simulink model "DebitPapillon_1"  (R2024b)
settings: Solver=FixedStepDiscrete  StartTime=0.0  StopTime=SimuPapStop  FixedStep=0.1  RelTol=1e-3  EnableMultiTasking=on
undefined symbols (not defined in the file): AirIntakeAirFlowTest, AirIntakeTemperatureTest, AirIntakeTimeTest, gam, Pamb, PcolPapTest, PRcrit, Rair, SectionPapTest, Tamb, TempsPapTest
settings Model: Creator=a030141  LastModifiedBy=ramse
settings SolverCC: AlgebraicLoopSolver=TrustRegion
settings DataIOCC: LimitDataPoints=on  SaveFormat=Array  SignalLoggingSaveFormat=ModelDataLogs  ReturnWorkspaceOutputs=off  SignalLoggingName=sigsOut
settings OptimizationCC: ReuseModelBlockBuffer=off  InitFltsAndDblsToZero=on  LifeSpan=inf
settings DebuggingCC: SaveWithParameterizedLinksMsg=none  UnderspecifiedInitializationDetection=Classic  MergeDetectMultiDrivingBlocksExec=none  SignalResolutionControl=TryResolveAllWithWarning  MultiTaskDSMMsg=warning  MultiTaskCondExecSysMsg=none  FcnCallInpInsideContextMsg=warning  UnconnectedInputMsg=warning  UnconnectedOutputMsg=warning  UnconnectedLineMsg=warning  SFUnexpectedBacktrackingDiag=warning  SFNoUnconditionalDefaultTransitionDiag=warning  SFExecutionAtInitializationDiag=none  ArithmeticOperatorsInVariantConditions=warning
settings HardwareCC: ProdBitPerPointer=32  ProdBitPerSizeT=32  ProdBitPerPtrDiffT=32  ProdLargestAtomicFloat=None  ProdIntDivRoundTo=Undefined  ProdEndianess=Unspecified  ProdWordSize=32  ProdHWDeviceType=32-bit Generic  TargetUnknown=on
settings ModelReferenceCC: PropagateSignalLabelsOutOfModel=off
settings RTWCC: GPUComputeCapability=3.5
settings CodeAppCC: StateflowObjectComments=on
settings GRTTargetCC: TargetFcnLib=ansi_tfl_tmw.mat  TargetLangStandard=C89/C90 (ANSI)  CombineOutputUpdateFcns=off  GRTInterface=on
settings ConfigComp: CovMetricSettings=dw  CovSaveCumulativeToWorkspaceVar=on  CovSaveSingleToWorkspaceVar=on

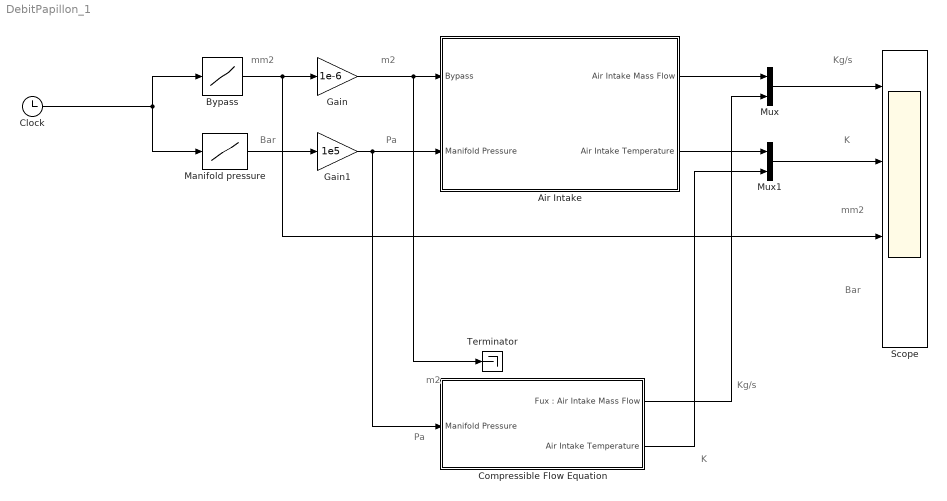
== system DebitPapillon_1 ==
  note: m2
  note: mm2
  note: Pa
  note: mm2
  note: K
  note: Kg/s
  note: Bar
  note: Bar
  note: m2
  note: Pa
  note: Kg/s
  note: K
  Air Intake : Subsystem
  Bypass : Lookup  InputValues=TempsPapTest  Table=SectionPapTest
  Clock : Clock
  Compressible Flow Equation : Subsystem
  Gain : Gain  Gain=1e-6  SaturateOnIntegerOverflow=on  OutDataTypeStr=Inherit: Same as input  ParamDataTypeStr=Inherit: Same as input
  Gain1 : Gain  Gain=1e5  SaturateOnIntegerOverflow=on  OutDataTypeStr=Inherit: Same as input  ParamDataTypeStr=Inherit: Same as input
  Manifold pressure : Lookup  InputValues=TempsPapTest  Table=PcolPapTest
  Mux : Mux  Inputs=2
  Mux1 : Mux  Inputs=2
  Scope : Scope  NumInputPorts=4
  Terminator : Terminator
  wires:
  Manifold pressure/1 -> Gain1/1
  Clock/1 -> Manifold pressure/1, Bypass/1
  Bypass/1 -> Gain/1, Scope/3
  Gain1/1 -> Compressible Flow Equation/1(Manifold Pressure), Air Intake/2(Manifold Pressure)
  Mux/1 -> Scope/1
  Mux1/1 -> Scope/2
  Compressible Flow Equation/2(Air Intake Temperature) -> Mux1/2
  Air Intake/1(Air Intake Mass Flow) -> Mux/1
  Air Intake/2(Air Intake Temperature) -> Mux1/1
  Compressible Flow Equation/1("Fux : Air Intake Mass Flow") -> Mux/2
  Gain/1 -> Terminator/1, Air Intake/1(Bypass)

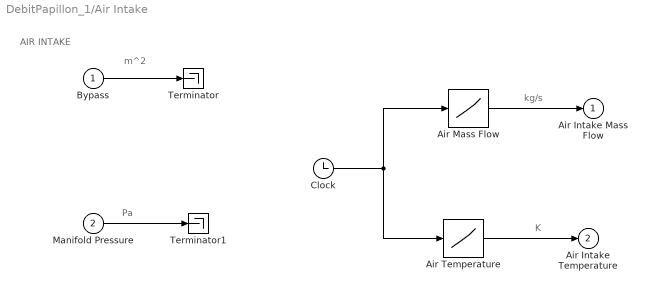
== system DebitPapillon_1/Air Intake ==
  note: AIR INTAKE
  note: m^2
  note: kg/s
  note: Pa
  note: K
  Bypass : Inport
  Manifold Pressure : Inport  Port=2
  Air Mass Flow : Lookup  InputValues=AirIntakeTimeTest  Table=AirIntakeAirFlowTest
  Air Temperature : Lookup  InputValues=AirIntakeTimeTest  Table=AirIntakeTemperatureTest
  Clock : Clock
  Terminator : Terminator
  Terminator1 : Terminator
  Air Intake Mass Flow : Outport
  Air Intake Temperature : Outport  Port=2
  wires:
  Air Mass Flow/1 -> Air Intake Mass Flow/1
  Manifold Pressure/1 -> Terminator1/1
  Bypass/1 -> Terminator/1
  Air Temperature/1 -> Air Intake Temperature/1
  Clock/1 -> Air Mass Flow/1, Air Temperature/1

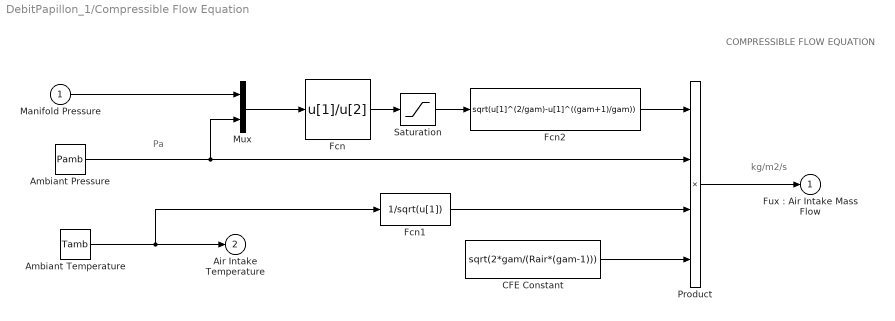
== system DebitPapillon_1/Compressible Flow Equation ==
  note: COMPRESSIBLE FLOW EQUATION
  note: Pa
  note: kg/m2/s
  Manifold Pressure : Inport
  Ambiant Pressure : Constant  Value=Pamb
  Ambiant Temperature : Constant  Value=Tamb
  "CFE Constant " : Constant  Value=sqrt(2*gam/(Rair*(gam-1)))
  Fcn : Fcn  Expr=u[1]/u[2]
  Fcn1 : Fcn  Expr=1/sqrt(u[1])
  Fcn2 : Fcn  Expr=sqrt(u[1]^(2/gam)-u[1]^((gam+1)/gam))
  Mux : Mux  Inputs=2
  Product : Product  Inputs=4  InputSameDT=on  SaturateOnIntegerOverflow=on  OutDataTypeStr=Inherit: Same as first input
  Saturation : Saturate  UpperLimit=1  LowerLimit=PRcrit
  "Fux : Air Intake Mass Flow" : Outport
  Air Intake Temperature : Outport  Port=2
  wires:
  Ambiant Pressure/1 -> Product/2, Mux/2
  Product/1 -> "Fux : Air Intake Mass Flow"/1
  "CFE Constant "/1 -> Product/4
  Fcn2/1 -> Product/1
  Saturation/1 -> Fcn2/1
  Fcn1/1 -> Product/3
  Fcn/1 -> Saturation/1
  Mux/1 -> Fcn/1
  Manifold Pressure/1 -> Mux/1
  Ambiant Temperature/1 -> Fcn1/1, Air Intake Temperature/1
